simulink model "DC_Motor_verified_"  (R2016b)
settings: Solver=VariableStepAuto  StartTime=0.0  StopTime=10.0  RelTol=1e-3
values from neighbouring files (symbols this model uses):
  param = zeros(3,1)    [parameter_estimation_script.m]
settings Model: Creator=dell  LastModifiedBy=dell

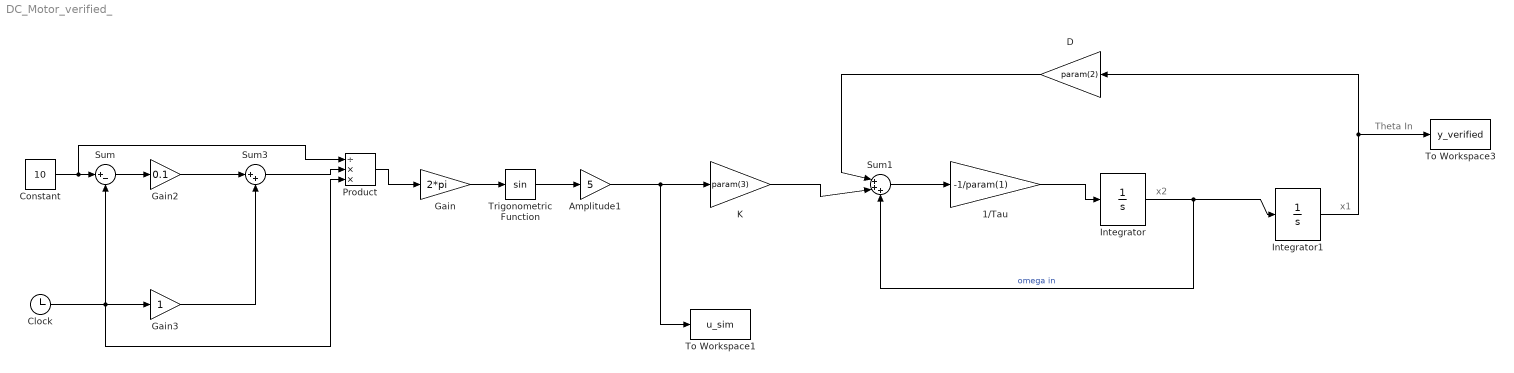
== system DC_Motor_verified_ ==
  note: Theta In
  note: x1
  note: x2
  1/Tau : Gain  Gain=-1/param(1)
  Amplitude1 : Gain  Gain=5
  Clock : Clock
  Constant : Constant  Value=10
  D : Gain  Gain=param(2)
  Gain : Gain  Gain=2*pi
  Gain2 : Gain  Gain=0.1
  Gain3 : Gain
  Integrator : Integrator
  Integrator1 : Integrator
  K : Gain  Gain=param(3)
  Product : Product  Inputs=/**
  Sum : Sum  Inputs=|+-
  Sum1 : Sum  Inputs=|+++
  Sum3 : Sum  Inputs=|++
  To Workspace1 : ToWorkspace  VariableName=u_sim  SaveFormat=Timeseries  SampleTime=-1
  To Workspace3 : ToWorkspace  VariableName=y_verified  SaveFormat=Timeseries  SampleTime=-1
  Trigonometric Function : Trigonometry
  wires:
  1/Tau/1 -> Integrator/1
  Constant/1 -> Product/1, Sum/1
  Product/1 -> Gain/1
  Gain3/1 -> Sum3/2
  Gain2/1 -> Sum3/1
  Sum3/1 -> Product/2
  Amplitude1/1 -> To Workspace1/1, K/1
  Integrator1/1 -> D/1, To Workspace3/1
  Integrator/1 -> Integrator1/1, Sum1/3  "omega in"
  Trigonometric Function/1 -> Amplitude1/1
  Gain/1 -> Trigonometric Function/1
  Clock/1 -> Product/3, Gain3/1, Sum/2
  Sum/1 -> Gain2/1
  D/1 -> Sum1/1
  K/1 -> Sum1/2
  Sum1/1 -> 1/Tau/1
